simulink model "model1"  (R2015a)
settings: Solver=ode1  StartTime=0.0  StopTime=15.0  FixedStep=0.01  RelTol=1e-3
settings Model: Creator=jleny  LastModifiedBy=jleny

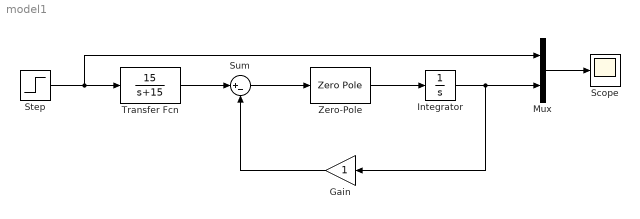
== system model1 ==
  Gain : Gain
  Integrator : Integrator
  Mux : Mux  Inputs=2
  Scope : Scope
      settings: SaveName=Y
  Step : Step  Time=2  Before=1  After=4  SampleTime=0
  Sum : Sum  Inputs=|+-
  Transfer Fcn : TransferFcn  Numerator=[15]  Denominator=[1 15]
  Zero-Pole : ZeroPole  Zeros=[-10]  Poles=[-1]
  wires:
  Step/1 -> Mux/1, Transfer Fcn/1
  Transfer Fcn/1 -> Sum/1
  Zero-Pole/1 -> Integrator/1
  Sum/1 -> Zero-Pole/1
  Gain/1 -> Sum/2
  Integrator/1 -> Gain/1, Mux/2
  Mux/1 -> Scope/1
